simulink model "testParseInC"  (R2015a)
settings: Solver=FixedStepDiscrete  StartTime=0.0  StopTime=Inf  FixedStep=0.001  RelTol=1e-3
undefined symbols (not defined in the file or in its folder): cbSpike
settings Model: SimulationMode=accelerator  Creator=djoshea  LastModifiedBy=djoshea
settings OptimizationCC: EnhancedBackFolding=on  SimCompilerOptimization=on
settings HardwareCC: ProdBitPerLong=64  ProdBitPerPointer=64  ProdIntDivRoundTo=Zero  ProdEndianess=LittleEndian  ProdWordSize=64  ProdHWDeviceType=Intel->x86-64  TargetBitPerLong=64  TargetBitPerPointer=64  TargetIntDivRoundTo=Zero  TargetEndianess=LittleEndian  TargetWordSize=64  TargetHWDeviceType=Intel->x86-64
settings SFSimCC: SimBuildMode=sf_nonincremental_build
settings RTWCC: SystemTargetFile=rtwin.tlc  TemplateMakefile=rtwin.tmf  Description=Simulink Desktop Real-Time  GenerateReport=on  RTWUseSimCustomCode=on  LaunchReport=on  RTWCompilerOptimization=on
settings CodeAppCC: MaxIdLength=95
settings RTWinTargetCC: TargetPreCompLibLocation=C:\Program Files\MATLAB\R2015a\toolbox\sldrt\lib\win64

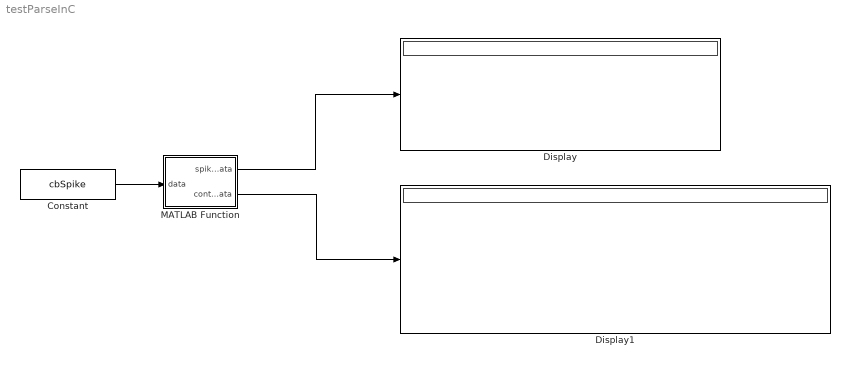
== system testParseInC ==
  Constant : Constant  Value=cbSpike
  Display : Display
  Display1 : Display
  MATLAB Function : MATLAB Function  TreatAsAtomicUnit=on
  wires:
  MATLAB Function/1(spikeData) -> Display/1
  Constant/1 -> MATLAB Function/1(data)
  MATLAB Function/2(contData) -> Display1/1

== matlab function testParseInC/MATLAB Function ==
  data: spikeData output; data input; contData output
function [spikeData, contData] = fcn(data)
%#codegen

coder.cinclude('C:\Users\djoshea\code\matudp\sandbox\cerebusParsing\cerebusParse.h');
coder.updateBuildInfo('addSourceFiles', 'C:\Users\djoshea\code\matudp\sandbox\cerebusParsing\cerebusParse.c');

% pp = coder.opaque('cbPKT_GENERIC*', 'NULL');
% pp = coder.ceval('cb_getPointer', coder.ref(data));

[pp, pBufferEnd] = CerebusParse.getPointers(data);

maxSpikes = 4;
spikeData = zeros(5, maxSpikes, 'int16');
nSpikes = uint32(0);

maxContSamples = 5;
maxChannels = 6;
contData = zeros(maxChannels, maxContSamples, 'int16');
nSamples = uint32(0);

nPackets = uint32(1);
while true
    if CerebusParse.isSpikePacket(pp)
        if nSpikes + uint32(1) > maxSpikes
            continue;
        end
        nSpikes = nSpikes + uint32(1);
        spikeData = CerebusParse.copySpikeWaveformToBufferColumn(pp, spikeData, nSpikes);

    elseif CerebusParse.isContinuousPacketForGroup(pp, uint8(5))
        if nSamples + uint32(1) > maxContSamples
            continue;
        end
        nSamples = nSamples + uint32(1);
        contData = CerebusParse.copyContinuousSamplesToBufferColumn(pp, contData, nSamples);
    end

    if ~CerebusParse.hasNext(pp, pBufferEnd)
        break;
    end
    pp = CerebusParse.getNext(pp);
    nPackets = nPackets + uint32(1);
end
